simulink model "zerInvS"  (Simulink 7.9)
settings: Solver=ode45  StartTime=0.0  StopTime=10.0  RelTol=1e-3
values from neighbouring files (symbols this model uses):
  c1 = 3    [zerInv.m]
  c2 = 1    [zerInv.m]
  c3 = 1    [zerInv.m]
libraries: simulink x1
settings Model: Creator=userk  LastModifiedBy=userk

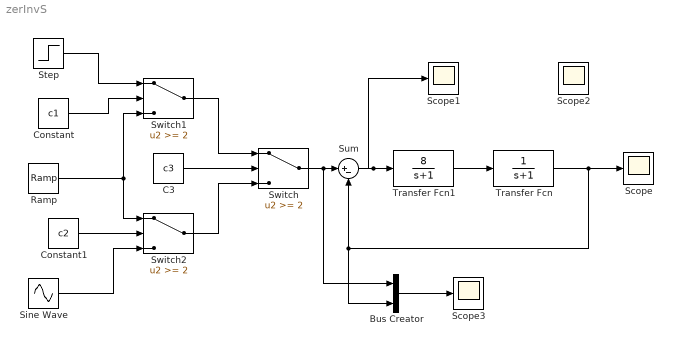
== system zerInvS ==
  Bus Creator : BusCreator  Inputs=2
  C3 : Constant  Value=c3
  Constant : Constant  Value=c1
  Constant1 : Constant  Value=c2
  Ramp : simulink/Sources/Ramp  slope=1  start=0  X0=0
  Scope{,1..3} (4 alike) : Scope
      Scope2 settings: SaveName=ScopeData2
      Scope3 settings: SaveName=ScopeData3
  Sine Wave : Sin  Frequency=3  SampleTime=0
  Step : Step  SampleTime=0
  Sum : Sum  Inputs=|+-
  Switch : Switch  Threshold=2
  Switch1 : Switch  Threshold=2
  Switch2 : Switch  Threshold=2
  Transfer Fcn : TransferFcn  Denominator=[1 1]
  Transfer Fcn1 : TransferFcn  Numerator=[8]  Denominator=[1 1]
  wires:
  Switch1/1 -> Switch/1
  C3/1 -> Switch/2
  Step/1 -> Switch1/1
  Constant/1 -> Switch1/2
  Ramp/1 -> Switch1/3, Switch2/1
  Constant1/1 -> Switch2/2
  Sine Wave/1 -> Switch2/3
  Switch2/1 -> Switch/3
  Transfer Fcn/1 -> Scope/1, Sum/2, Bus Creator/2
  Transfer Fcn1/1 -> Transfer Fcn/1
  Sum/1 -> Scope1/1, Transfer Fcn1/1
  Switch/1 -> Sum/1, Bus Creator/1
  Bus Creator/1 -> Scope3/1
